simulink model "SystemModel"  (R2026a)
settings: Solver=FixedStepDiscrete  StopTime=inf  FixedStep=ts_system  EnableMultiTasking=on
StartFcn:
  | Simulink.sdi.setRecordData(false);
undefined symbols (not defined in the file): Battery, BCE12, BCE_Set_init, BMS_Controller_State, Cell10_P, Cell11_P, Cell12_P, Cell1_N, Cell1_P, Cell2_P, Cell3_P, Cell4_P, Cell5_P, Cell6_P, Cell7_P, Cell8_P, Cell9_P, Cell_Temperatures, Cell_Voltages, Charging_State, currentFactor, CV_Gain, Device_01, DiscIntNeverNeededParam, I_cc, MaxCellVoltThrsld, noCurrent, Ns_Module, NumModules, OverCellVoltageLimit, sg_bce, SOCInit, SRE, ts_controller, ts_system, UnderCellVoltageLimit, voltThreshold
libraries: slrealtimeethercatlib x99, fl_lib x65, nesl_utility x43, simulink x23, slrealtimeutilitieslib x13, sl_discontinuities x13, dspstat3 x12, canmsglib x11, speedgoatlib_IO611 x9, batt_lib x3, sharedTrackingLibrary x2, BatteryModuleLibrary_12Cells_lib x1
(part 3 of 6)

== system SystemModel/BMS/HIL ==
  note: Terminate the "Cells" Simscape Bus
  State_Request : Inport  OutDataTypeStr=Enum: SRE  PortDimensions=1
  Sensor_Values : Inport  Port=2
  Bus Creator : BusCreator  Inputs=4  OutDataTypeStr=Bus: Controller_Info  NonVirtualBus=on
      settings: InheritFromInputs=off
  Bus Creator1 : BusCreator  Inputs=4  OutDataTypeStr=Bus: Controller_Output  NonVirtualBus=on
      settings: InheritFromInputs=off
  Cell Monitoring Unit : Subsystem
  Controller : Subsystem  VariantControl=Ns_Module == 12
  Rate Transition : RateTransition  InitialCondition=struct('Cell_Voltages',3.7*ones(1,Ns_Module),'Cell_Temperatures',298.15*ones(1,Ns_Module),'Pack_Current',0,'Pack_Voltage',3.7*Ns_Module)  OutPortSampleTime=ts_controller
  Rate Transition1 : RateTransition  InitialCondition=SRE.Standby  OutPortSampleTime=ts_controller
  Simscape Bus : SimscapeBus
  Cells : PMIOPort  Side=Left
  Controller_Info : Outport
  Controller_Output : Outport  Port=2  OutDataTypeStr=Bus: Controller_Output  VectorParamsAs1DForOutWhenUnconnected=off  BusOutputAsStruct=on
  wires:
  Bus Creator/1 -> Controller_Info/1  "Controller_Info"
  Bus Creator1/1 -> Controller_Output/1  "Controller_Output"
  [Bal_Cmd_Controller] -> Cell Monitoring Unit/1(Bal_Cmd_Controller)
  Cell Monitoring Unit/1(Bal_Cmd) -> Bus Creator1/4
  Rate Transition/1 -> Cell Monitoring Unit/2(Sensor_Values)
  Cell Monitoring Unit/2(Sensor Values) -> Controller/1(Sensor_Values)
  Rate Transition1/1 -> Controller/2(State_Request)
  Controller/1(BMS_Faults) -> Bus Creator/1
  Controller/2(Charging_State) -> Bus Creator/2
  Controller/3(BMS_State) -> Bus Creator/3
  Controller/4(SOC) -> Bus Creator/4
  Controller/5(Discharge_Current_Limit) -> Bus Creator1/1
  Controller/6(Charge_Current_Limit) -> Bus Creator1/2
  Controller/7(Charge_Current_Req) -> Bus Creator1/3
  Controller/8(Bal_Cmd) -> [Bal_Cmd_Controller]
  State_Request/1 -> Rate Transition1/1
  Sensor_Values/1 -> Rate Transition/1
  connections:
  Simscape Bus/RConn1 -- Cells/RConn1

== system SystemModel/BMS/MIL ==
  State_Request : Inport  OutDataTypeStr=Enum: SRE  PortDimensions=1
  Sensor_Values : Inport  Port=2  OutDataTypeStr=Bus: Sensor_Values  BusOutputAsStruct=on
  Bus Creator : BusCreator  Inputs=4  OutDataTypeStr=Bus: Controller_Info  NonVirtualBus=on
      settings: InheritFromInputs=off
  Bus Creator1 : BusCreator  Inputs=4  OutDataTypeStr=Bus: Controller_Output  NonVirtualBus=on
      settings: InheritFromInputs=off
  Cell Monitoring Unit : Subsystem
  Controller : Subsystem
  Rate Transition : RateTransition  InitialCondition=struct('Cell_Voltages',3.7*ones(1,Ns_Module),'Cell_Temperatures',298.15*ones(1,Ns_Module),'Pack_Current',0,'Pack_Voltage',3.7*Ns_Module)  OutPortSampleTime=ts_controller
  Rate Transition1 : RateTransition  InitialCondition=SRE.Standby  OutPortSampleTime=ts_controller
  Cells : PMIOPort  Side=Left
  Controller_Info : Outport
  Controller_Output : Outport  Port=2  OutDataTypeStr=Bus: Controller_Output  VectorParamsAs1DForOutWhenUnconnected=off  BusOutputAsStruct=on
  wires:
  Bus Creator/1 -> Controller_Info/1  "Controller_Info"
  Bus Creator1/1 -> Controller_Output/1  "Controller_Output"
  State_Request/1 -> Rate Transition1/1
  Controller/1(Faults) -> Bus Creator/1
  Controller/2(Charging_State) -> Bus Creator/2  "Charging_State"
  Controller/3(BMS_Controller_State) -> Bus Creator/3  "BMS_State"
  Controller/4(SOC) -> Bus Creator/4
  Controller/5(Discharge_Current_Limit) -> Bus Creator1/1
  Controller/6(Charge_Current_Limit) -> Bus Creator1/2
  Controller/7(Charge_Current_Req) -> Bus Creator1/3
  Controller/8(Bal_Cmd) -> [Bal_Cmd_Controller]
  [Bal_Cmd_Controller] -> Cell Monitoring Unit/1(Bal_Cmd_Controller)
  Sensor_Values/1 -> Rate Transition/1
  Cell Monitoring Unit/1(Bal_Cmd) -> Bus Creator1/4
  Cell Monitoring Unit/2(Sensor Values) -> Controller/1(Sensor_Values)
  Rate Transition1/1 -> Controller/2(State_Request)
  Rate Transition/1 -> Cell Monitoring Unit/2(Sensor_Values)
  connections:
  Cells/RConn1 -- Cell Monitoring Unit/LConn1

== system SystemModel/Battery/Battery Pack ==
  Ambient_Temperature : Inport
  Short_Circuits : Inport  Port=2
  12-Cell : Subsystem  VariantControl=Ns_Module == 12
  Batt+ : PMIOPort  Side=Right
  Batt- : PMIOPort  Port=2  Side=Right
  Cells : PMIOPort  Port=3  Side=Right
  Cell_Voltages : Outport
  Cell_Temperatures : Outport  Port=2
  Cell_SOCs : Outport  Port=3
  wires:
  Ambient_Temperature/1 -> 12-Cell/1(Ambient_Temperature)
  Short_Circuits/1 -> 12-Cell/2(Short_Circuits)
  12-Cell/1(Cell_Voltages) -> Cell_Voltages/1
  12-Cell/2(Cell_Temperatures) -> Cell_Temperatures/1
  12-Cell/3(Cell_SOCs) -> Cell_SOCs/1
  connections:
  12-Cell/RConn1 -- Batt+/RConn1
  12-Cell/RConn2 -- Batt-/RConn1
  12-Cell/RConn3 -- Cells/RConn1

== system SystemModel/Battery/Bypass ==
  IN : Inport
  Bus Assignment : BusAssignment  AssignedSignals=Cell_Voltages,Cell_Temperatures
  Bus Selector : BusSelector  OutputSignals=Cell_Voltages,Cell_Temperatures
  Bypass Values : Subsystem
  Data Type Conversion{,1..3} (4 alike) : DataTypeConversion  OutDataTypeStr=single  SaturateOnIntegerOverflow=off  RndMeth=Floor
  OUT : Outport
  wires:
  IN/1 -> Bus Assignment/1, Bus Selector/1
  Bus Assignment/1 -> OUT/1
  [Cell_Voltages_OUT] -> Data Type Conversion/1
  [Cell_Temperatures_OUT] -> Data Type Conversion1/1
  Bus Selector/1 -> [Cell_Voltages_IN]  "<Cell_Voltages>"
  Bus Selector/2 -> [Cell_Temperatures_IN]  "<Cell_Temperatures>"
  Data Type Conversion/1 -> Bus Assignment/2
  Data Type Conversion1/1 -> Bus Assignment/3
  Data Type Conversion2/1 -> [Cell_Voltages_OUT]
  Data Type Conversion3/1 -> [Cell_Temperatures_OUT]
  [Cell_Voltages_IN] -> Bypass Values/1(Input_Voltages)
  [Cell_Temperatures_IN] -> Bypass Values/2(Input_Temperatures)
  Bypass Values/1(Output_Voltages) -> Data Type Conversion2/1
  Bypass Values/2(Output_Temperatures) -> Data Type Conversion3/1
  [Broken_Wires_User] -> Bypass Values/3(Broken_Wire)

== system SystemModel/Battery/Electrical Interface ==
  Current_Request : Inport
  Controlled Current Source : fl_lib/Electrical/Electrical Sources/Controlled Current Source
  Current Sensor : fl_lib/Electrical/Electrical Sensors/Current Sensor
  Data Type Conversion : DataTypeConversion  OutDataTypeStr=double  SaturateOnIntegerOverflow=off  RndMeth=Floor
  Electrical Reference : fl_lib/Electrical/Electrical Elements/Electrical Reference
  PS-Simulink Converter : nesl_utility/PS-Simulink Converter  PhysicalDomain=network_engine_domain  SubClassName=ps_output  LeftPortType=input  RightPortType=output  PseudoPeriodic=off  Frequencies=[]  VectorFormat=inherit  Unit=inherit  AffineConversion=off
  PS-Simulink Converter1 : nesl_utility/PS-Simulink Converter  PhysicalDomain=network_engine_domain  SubClassName=ps_output  LeftPortType=input  RightPortType=output  PseudoPeriodic=off  Frequencies=[]  VectorFormat=inherit  Unit=inherit  AffineConversion=off
  Simulink-PS Converter3 : nesl_utility/Simulink-PS Converter  PhysicalDomain=network_engine_domain  SubClassName=ps_input  LeftPortType=input  RightPortType=output  PseudoPeriodic=off  Frequencies=[]  NoiseDistribution=none  NoiseParameters=[]  Unit=1  AffineConversion=off  FilteringAndDerivatives=zero  SimscapeFilterOrder=1  InputFilterTimeConstant=0.001  UdotUserProvided=1
  Solver Configuration : nesl_utility/Solver Configuration  PhysicalDomain=network_engine_domain  SubClassName=solver  LeftPortType=input  RightPortType=generic  Tones=[]  Harmonics=[]  SimulateNoise=off  Profile=off  UseLocalSampling=off  EnableSwitchedLinearOptims=on  FrequencyDomain=off  UseCCode=off  RelTol=0.001  AbsTol=0.001  MinStep=1e-09  ToWorkspace=off  RevertToSquareIcSolve=off  NumHomotopyIterations=100  PhasorMode=off  PhasorModeNumHarmonics=1  ConsistencySolver=NEWTON_XTOL_AFTER_FTOL  CanonicalOrdering=UNORDERED  OptimizeIntermediates=UNOPTIMIZED  IndexReductionMethod=DerivativeReplacement  DoDC=off  ResidualTolerance=1e-09  ConsistencyTolSource=GLOBAL  ConsistencyAbsTol=0.001  ConsistencyRelTol=0.001  ConsistencyTolFactor=1e-09  UseLocalSolver=on  LocalSolverChoice=NE_BACKWARD_EULER_ADVANCER  ResolveIndetEquations=on  FunctionEvalNumThread=1  LocalSolverSampleTime=ts_system  DoFixedCost=on  MaxNonlinIter=3  MaxModeIter=2  ComputeImpulses=off  ImpulseIterations=2  LinearAlgebra=auto  LinearAlgebraNumThread=0  EquationFormulation=NE_TIME_EF  DelaysMemoryBudget=1024  AutomaticFiltering=on  FilteringTimeConstant=0.001  PartitionStorageMethod=AS_NEEDED  PartitionMemoryBudget=1024  PartitionMethod=ROBUST  MultibodyUseLocalSolver=off  MultibodyLocalSolverChoice=ODE1  MultibodyLocalSolverSampleTime=0.001
  Voltage Sensor7 : fl_lib/Electrical/Electrical Sensors/Voltage Sensor
      settings: LibrarySourceBlock=BatteryPack_lib/CellMonitoringUnit/Voltage Sensor1
  Batt+ : PMIOPort  Side=Left
  Batt- : PMIOPort  Port=2  Side=Left
  Pack_Current : Outport
  Pack_Voltage : Outport  Port=2
  wires:
  Current_Request/1 -> Data Type Conversion/1
  PS-Simulink Converter1/1 -> Pack_Current/1
  PS-Simulink Converter/1 -> Pack_Voltage/1
  Data Type Conversion/1 -> Simulink-PS Converter3/1
  connections:
  Controlled Current Source/LConn1 -- Voltage Sensor7/LConn1 -- Batt+/RConn1
  Current Sensor/RConn2 -- Solver Configuration/RConn1 -- Electrical Reference/LConn1 -- Controlled Current Source/RConn2
  PS-Simulink Converter1/LConn1 -- Current Sensor/RConn1
  Simulink-PS Converter3/RConn1 -- Controlled Current Source/RConn1
  Batt-/RConn1 -- Voltage Sensor7/RConn2 -- Current Sensor/LConn1
  Voltage Sensor7/RConn1 -- PS-Simulink Converter/LConn1

== system SystemModel/Battery/HW Interface ==
  Sensor_Values_Sim : Inport
  BCE - HIL : Subsystem  VariantControl=strcmp(get_param([bdroot '/Instrumentation/Simulation_Profile_Value'], 'Value'),'1') && Ns_Module == 12
  MIL : Subsystem  VariantControl=strcmp(get_param([bdroot '/Instrumentation/Simulation_Profile_Value'], 'Value'),'0')
  Cells_IN : PMIOPort  Side=Left
  Cells_OUT : PMIOPort  Port=2  Side=Right
  Sensor_Values_Real : Outport

== system SystemModel/Instrumentation/Celsius_to_Kelvin ==
  C : Inport
  Add : Sum
  Constant4 : Constant  Value=273.15
  K : Outport
  wires:
  Constant4/1 -> Add/2
  C/1 -> Add/1
  Add/1 -> K/1

== system SystemModel/Instrumentation/Current Control ==
  Current_Request_User : Inport
  Current_Request_User_Bypass : Inport  Port=2
  Controller_Info : Inport  Port=3
  Controller_Output : Inport  Port=4
  Bus Selector : BusSelector  OutputSignals=Charge_Current_Limit,Discharge_Current_Limit
  Bus Selector1 : BusSelector  OutputSignals=BMS_State
  Compare To Constant : simulink/Logic and Bit Operations/Compare To Constant  relop===  const=BMS_Controller_State.BMS_Fault  OutDataTypeStr=uint8
  Current_Req : Constant  Value=0  SampleTime=ts_controller
  Saturation Dynamic : sl_discontinuities/Saturation Dynamic  OutMin=[]  OutMax=[]  OutDataTypeStr=Inherit: Same as second input  OutDataType=fixdt(1, 16)  OutScaling=2^-10  DoSatur=off
  Switch : Switch  Criteria=u2 > Threshold  SaturateOnIntegerOverflow=off  InputSameDT=off
  Switch1 : Switch  Criteria=u2 > Threshold  SaturateOnIntegerOverflow=off  InputSameDT=off
  Current_Request : Outport
  wires:
  Current_Request_User/1 -> Saturation Dynamic/2, Switch1/1
  Controller_Output/1 -> Bus Selector/1
  Bus Selector/1 -> Saturation Dynamic/1  "<Charge_Current_Limit>"
  Bus Selector/2 -> Saturation Dynamic/3  "<Discharge_Current_Limit>"
  Current_Req/1 -> Switch/1
  Saturation Dynamic/1 -> Switch/3
  Controller_Info/1 -> Bus Selector1/1
  Bus Selector1/1 -> Compare To Constant/1  "<BMS_State>"
  Switch1/1 -> Current_Request/1
  Switch/1 -> Switch1/3
  Current_Request_User_Bypass/1 -> Switch1/2
  Compare To Constant/1 -> Switch/2

== system SystemModel/Instrumentation/Instrumented Signals ==
  Controller_Output : Inport
  Controller_Info : Inport  Port=2
  Sensor_Values : Inport  Port=3
  Balancing_Currents : Inport  Port=4
  Cells_SOCs : Inport  Port=5
  12-Cell : Subsystem  VariantControl=Ns_Module == 12
  Short-Circuits : Outport
  Broken_Wires : Outport  Port=2
  wires:
  Controller_Output/1 -> 12-Cell/1(Controller_Output)
  Controller_Info/1 -> 12-Cell/2(Controller_Info)
  Sensor_Values/1 -> 12-Cell/3(Sensor_Values)
  Balancing_Currents/1 -> 12-Cell/4(Balancing_Currents)
  Cells_SOCs/1 -> 12-Cell/5(Cells_SOCs)
  12-Cell/1(Short-Circuits) -> Short-Circuits/1
  12-Cell/2(Broken_Wires) -> Broken_Wires/1

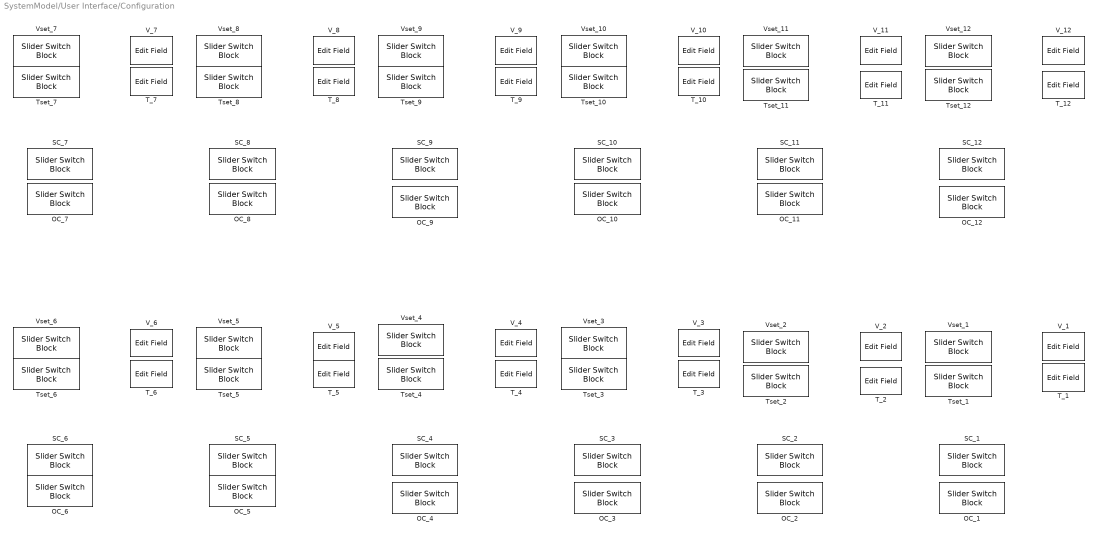
== system SystemModel/User Interface/Configuration ==
  OC_{1..12} (12 alike) : SliderSwitchBlock  LabelPosition=Hide
  SC_{1..12} (12 alike) : SliderSwitchBlock  LabelPosition=Hide
  T_{1..12} (12 alike) : EditField  LabelPosition=Hide  ShowInitialText=on  Alignment=Center
  Tset_{1..12} (12 alike) : SliderSwitchBlock  LabelPosition=Hide
  V_{1..12} (12 alike) : EditField  LabelPosition=Hide  ShowInitialText=on  Alignment=Center
  Vset_{1..12} (12 alike) : SliderSwitchBlock  LabelPosition=Hide

== system SystemModel/BMS/HIL/Cell Monitoring Unit ==
  Bal_Cmd_Controller : Inport
  Sensor_Values : Inport  Port=2
  Bal_Cmd : Outport
  Sensor Values : Outport  Port=2
  wires:
  Sensor_Values/1 -> Sensor Values/1
  Bal_Cmd_Controller/1 -> Bal_Cmd/1  "Bal_Cmd"

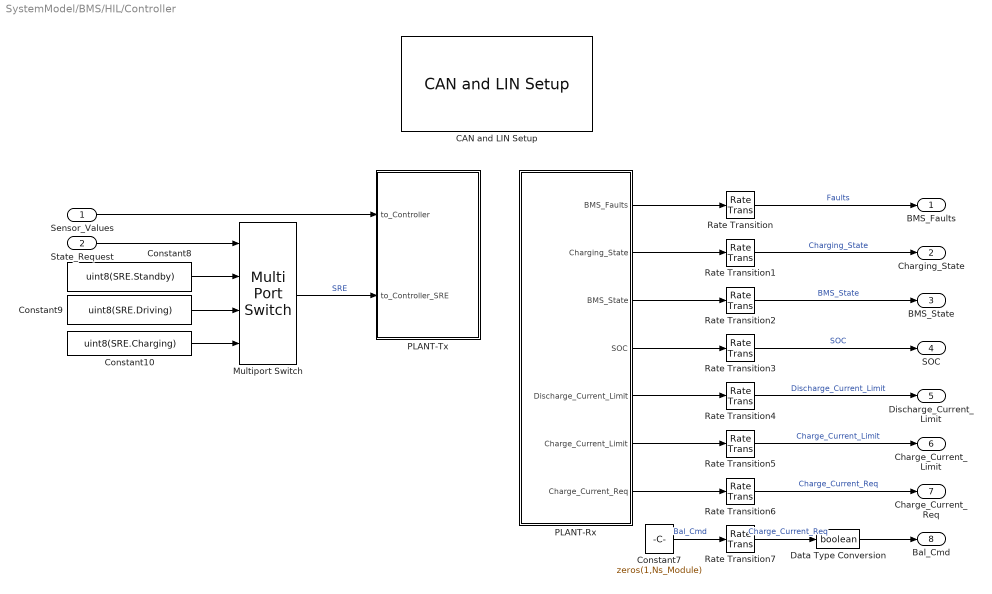
== system SystemModel/BMS/HIL/Controller ==
  Sensor_Values : Inport  OutDataTypeStr=Bus: Sensor_Values  BusOutputAsStruct=on
  State_Request : Inport  Port=2  OutDataTypeStr=Enum: SRE  PortDimensions=1
  "CAN and LIN Setup " : speedgoatlib_IO611/CAN and LIN Setup   moduleInitValues="[611    1    1   -1   -1]"  id=1  moduleType=IO611  pciSlot=-1  canChn1=CAN (HS)  canChn2=CAN (HS)  canChn3=Disabled  canChn4=Disabled  linChn1=Disabled  linChn2=Disabled  canInitStructArray=[]  canTermStructArray=[]  canChn1InitValues="[2   2   1  31   8   2   1   5   2]"  arbBdrChn1=1.0 MBaud  arbManBdrChn1=[2,1,31,8]  fdBdrChn1=5.0 MBaud  fdManBdrChn1=[2,1,5,2]  canChn2InitValues="[2   2   1  31   8   2   1   5   2]"  arbBdrChn2=1.0 MBaud  arbManBdrChn2=[2,1,31,8]  fdBdrChn2=5.0 MBaud  fdManBdrChn2=[2,1,5,2]  canChn3InitValues="[1   2   1  31   8   2   1   5   2]"  arbBdrChn3=1.0 MBaud  arbManBdrChn3=[2,1,31,8]  fdBdrChn3=5.0 MBaud  fdManBdrChn3=[2,1,5,2]  canChn4InitValues="[1   2   1  31   8   2   1   5   2]"  arbBdrChn4=1.0 MBaud  arbManBdrChn4=[2,1,31,8]  fdBdrChn4=5.0 MBaud  fdManBdrChn4=[2,1,5,2]  bdrLIN1=19200  linChn1InitValues="[1  19200]"  bdrLIN2=19200  linChn2InitValues="[1  19200]"
      settings: LibrarySourceBlock=speedgoatlib_CANLIN_OfA2/CAN and LIN Setup
  Constant10 : Constant  Value=uint8(SRE.Charging)
  Constant7 : Constant  Value=zeros(1,Ns_Module)
  Constant8 : Constant  Value=uint8(SRE.Standby)
  Constant9 : Constant  Value=uint8(SRE.Driving)
  Data Type Conversion : DataTypeConversion  OutDataTypeStr=boolean  SaturateOnIntegerOverflow=off  RndMeth=Floor
  Multiport Switch : MultiPortSwitch  DataPortOrder=Specify indices  DataPortIndices={SRE.Standby, SRE.Driving, SRE.Charging}  SaturateOnIntegerOverflow=off  InputSameDT=off
  PLANT-Rx : Subsystem  TreatAsAtomicUnit=on
  PLANT-Tx : Subsystem
  Rate Transition : RateTransition  InitialCondition=struct('OverCurrent',0,'HighTemp',0,'LowTemp',0,'OverVolt',0,'UnderVolt',0)  OutPortSampleTime=ts_controller
  Rate Transition1 : RateTransition  InitialCondition=Charging_State.Init  OutPortSampleTime=ts_controller
  Rate Transition2 : RateTransition  InitialCondition=BMS_Controller_State.BMS_Idle  OutPortSampleTime=ts_controller
  Rate Transition3 : RateTransition  InitialCondition=[0, 0, 0]  OutPortSampleTime=ts_controller
  Rate Transition4 : RateTransition  InitialCondition=-100  OutPortSampleTime=ts_controller
  Rate Transition5 : RateTransition  InitialCondition=40  OutPortSampleTime=ts_controller
  Rate Transition6 : RateTransition  OutPortSampleTime=ts_controller
  Rate Transition7 : RateTransition  OutPortSampleTime=ts_controller
  BMS_Faults : Outport
  Charging_State : Outport  Port=2
  BMS_State : Outport  Port=3
  SOC : Outport  Port=4
  Discharge_Current_Limit : Outport  Port=5
  Charge_Current_Limit : Outport  Port=6
  Charge_Current_Req : Outport  Port=7
  Bal_Cmd : Outport  Port=8
  wires:
  Constant7/1 -> Rate Transition7/1  "Bal_Cmd"
  Constant9/1 -> Multiport Switch/3
  Constant10/1 -> Multiport Switch/4
  Constant8/1 -> Multiport Switch/2
  State_Request/1 -> Multiport Switch/1
  PLANT-Rx/1(BMS_Faults) -> Rate Transition/1
  PLANT-Rx/7(Charge_Current_Req) -> Rate Transition6/1
  PLANT-Rx/6(Charge_Current_Limit) -> Rate Transition5/1
  PLANT-Rx/5(Discharge_Current_Limit) -> Rate Transition4/1
  PLANT-Rx/4(SOC) -> Rate Transition3/1
  PLANT-Rx/3(BMS_State) -> Rate Transition2/1
  PLANT-Rx/2(Charging_State) -> Rate Transition1/1
  Rate Transition/1 -> BMS_Faults/1  "Faults"
  Rate Transition1/1 -> Charging_State/1  "Charging_State"
  Rate Transition2/1 -> BMS_State/1  "BMS_State"
  Rate Transition3/1 -> SOC/1  "SOC"
  Rate Transition4/1 -> Discharge_Current_Limit/1  "Discharge_Current_Limit"
  Rate Transition5/1 -> Charge_Current_Limit/1  "Charge_Current_Limit"
  Rate Transition6/1 -> Charge_Current_Req/1  "Charge_Current_Req"
  Data Type Conversion/1 -> Bal_Cmd/1
  Rate Transition7/1 -> Data Type Conversion/1  "Charge_Current_Req"
  Sensor_Values/1 -> PLANT-Tx/1(to_Controller)
  Multiport Switch/1 -> PLANT-Tx/2(to_Controller_SRE)  "SRE"

== system SystemModel/BMS/MIL/Cell Monitoring Unit ==
  Bal_Cmd_Controller : Inport
  Sensor_Values : Inport  Port=2
  Balancing_Circuit : Subsystem
  Feedback Unit : UnitDelay  InitialCondition=struct('Cell_Voltages',3.6*ones(1, Ns_Module*NumModules),'Cell_Temperatures',293.15*ones(1,Ns_Module*NumModules),'Pack_Current',0,'Pack_Voltage',3.6*Ns_Module*NumModules)  SampleTime=-1
  Rate Transition1 : RateTransition  InitialCondition=zeros(1,Ns_Module)  OutPortSampleTime=ts_system
  Cells : PMIOPort  Side=Left
  Bal_Cmd : Outport
  Sensor Values : Outport  Port=2
  tag scope: Balancing_Currents=global
  wires:
  Feedback Unit/1 -> Sensor Values/1
  Sensor_Values/1 -> Feedback Unit/1
  Bal_Cmd_Controller/1 -> Bal_Cmd/1, Rate Transition1/1
  Rate Transition1/1 -> Balancing_Circuit/1(Bal_Cmd_Controller)
  Balancing_Circuit/1(Balancing_Currents) -> [Balancing_Currents]
  connections:
  Balancing_Circuit/LConn1 -- Cells/RConn1

== system SystemModel/BMS/MIL/Controller ==
  Sensor_Values : Inport  OutDataTypeStr=Bus: Sensor_Values  BusOutputAsStruct=on
  State_Request : Inport  Port=2  OutDataTypeStr=Enum: SRE  PortDimensions=1
  BMS State Machine : Subsystem
  Balancing Logic : Subsystem
  Constant : Constant
  Current Calculations : Subsystem
  SOC Calculation : Subsystem
  Faults : Outport
  Charging_State : Outport  Port=2
  BMS_Controller_State : Outport  Port=3
  SOC : Outport  Port=4
  Discharge_Current_Limit : Outport  Port=5
  Charge_Current_Limit : Outport  Port=6
  Charge_Current_Req : Outport  Port=7
  Bal_Cmd : Outport  Port=8
  wires:
  SOC Calculation/1(SOC) -> SOC/1
  Current Calculations/1(Discharge_Current_Limit) -> Discharge_Current_Limit/1, BMS State Machine/1(Discharge_Current_Limit)
  BMS State Machine/2(Faults) -> Faults/1
  BMS State Machine/1(Charge_Current_Req) -> Charge_Current_Req/1
  Sensor_Values/1 -> Balancing Logic/2(Sensor_Values), SOC Calculation/2(Sensor_Values), BMS State Machine/4(Sensor_Values), Current Calculations/1(BMS_Input)
  BMS State Machine/4(BMS_State) -> BMS_Controller_State/1, Balancing Logic/1(BMS_State), SOC Calculation/1(BMS_State)
  Current Calculations/2(Charge_Current_Limit) -> Charge_Current_Limit/1, BMS State Machine/2(Charge_Current_Limit)
  Balancing Logic/1(Bal_Cmd) -> Bal_Cmd/1  "Bal_Cmd"
  State_Request/1 -> BMS State Machine/3(State_Request)
  Constant/1 -> BMS State Machine/5(Fault_Reset_Enable)
  BMS State Machine/3(Charging_State) -> Charging_State/1

== system SystemModel/Battery/Battery Pack/12-Cell ==
  Ambient_Temperature : Inport
  Short_Circuits : Inport  Port=2
  Controlled Temperature Source : fl_lib/Thermal/Thermal Sources/Controlled Temperature Source
      settings: LibrarySourceBlock=|
      | BatteryPack_lib/CellModule1TC/Controlled
      | Temperature Source
  Delay : Delay
  Faults : Subsystem
  Module1 : BatteryModuleLibrary_12Cells_lib/Module1  BatteryCapacityCell=27 A*hr  ExtrapolationMethodCell=simscape.enum.extrapolation.nearest  SOCBreakpointsCell=[0, .1, .25, .5, .75, .9, 1]  TemperatureBreakpointsCell=[278, 293, 313] K  OpenCircuitVoltageThermalCell=[3.49, 3.5, 3.51; 3.55, 3.57, 3.56; 3.62, 3.63, 3.64; 3.71, 3.71, 3.72; 3.91, 3.93, 3.94; 4.07, 4.08, 4.08; 4.19, 4.19, 4.19] V  VoltageRangeCell=[0, inf] V  ResistanceSOCBreakpointsCell=[0, .1, .25, .5, .75, .9, 1]  ResistanceTemperatureBreakpointsCell=[278, 293, 313] K  R0ThermalCell=[.0117, .0085, .009; .011, .0085, .009; .0114, .0087, .0092; .0107, .0082, .0088; .0107, .0083, .0091; .0113, .0085, .0089; .0116, .0085, .0089] Ohm  BatteryThermalMassCell=100 J/K  AmbientResistance=25 K/W  P=1  S=12  socCell_specify=off  socCell_priority=High  socCell=repmat(1, 12, 1)  socCell_nominal_specify=off  socCell_nominal_value=1  socCell_nominal_unit=1  numCycles_specify=off  numCycles_priority=High  numCycles=repmat(0, 12, 1)  numCycles_nominal_specify=off  numCycles_nominal_value=1  numCycles_nominal_unit=1  batteryVoltage_specify=off  batteryVoltage_priority=None  batteryVoltage=repmat(0, 12, 1) V  batteryVoltage_nominal_specify=off  batteryVoltage_nominal_value=1  batteryVoltage_nominal_unit=V  batteryCurrent_specify=off  batteryCurrent_priority=None  batteryCurrent=repmat(0, 12, 1) A  batteryCurrent_nominal_specify=off  batteryCurrent_nominal_value=1  batteryCurrent_nominal_unit=A  batteryTemperature_specify=off  batteryTemperature_priority=High  batteryTemperature=repmat(298.15, 12, 1) K  batteryTemperature_nominal_specify=off  batteryTemperature_nominal_value=1  batteryTemperature_nominal_unit=K  vParallelAssembly_specify=off  vParallelAssembly_priority=None  vParallelAssembly=repmat(0, 12, 1) V  vParallelAssembly_nominal_specify=off  vParallelAssembly_nominal_value=1  vParallelAssembly_nominal_unit=V  socParallelAssembly_specify=off  socParallelAssembly_priority=None  socParallelAssembly=repmat(1, 12, 1)  socParallelAssembly_nominal_specify=off  socParallelAssembly_nominal_value=1  socParallelAssembly_nominal_unit=1
  PS-Simulink Converter : nesl_utility/PS-Simulink Converter  PhysicalDomain=network_engine_domain  SubClassName=ps_output  LeftPortType=input  RightPortType=output  PseudoPeriodic=off  Frequencies=[]  VectorFormat=inherit  Unit=inherit  AffineConversion=off
  Passive Balancing Interface : batt_lib/HIL/Passive Balancing Interface  balancingCircuitCount=12
  Probe : SimscapeProbe  BoundBlock=23330  Variables={batteryTemperature, socParallelAssembly}
  Simulink-PS Converter : nesl_utility/Simulink-PS Converter  PhysicalDomain=network_engine_domain  SubClassName=ps_input  LeftPortType=input  RightPortType=output  PseudoPeriodic=off  Frequencies=[]  NoiseDistribution=none  NoiseParameters=[]  Unit=1  AffineConversion=off  FilteringAndDerivatives=provide  SimscapeFilterOrder=1  InputFilterTimeConstant=0.001  UdotUserProvided=0
  Simulink-PS Converter1 : nesl_utility/Simulink-PS Converter  PhysicalDomain=network_engine_domain  SubClassName=ps_input  LeftPortType=input  RightPortType=output  PseudoPeriodic=off  Frequencies=[]  NoiseDistribution=none  NoiseParameters=[]  Unit=1  AffineConversion=off  FilteringAndDerivatives=provide  SimscapeFilterOrder=1  InputFilterTimeConstant=0.001  UdotUserProvided=0
      settings: LibrarySourceBlock=|
      | BatteryPack_lib/CellModule1TC/Simulink-PS
      | Converter1
  Batt+ : PMIOPort  Side=Right
  Batt- : PMIOPort  Port=2  Side=Right
  Cells : PMIOPort  Port=3  Side=Right
  Cell_Voltages : Outport
  Cell_Temperatures : Outport  Port=2
  Cell_SOCs : Outport  Port=3
  wires:
  [Balancing_Currents] -> Delay/1
  Probe/1 -> Cell_Temperatures/1
  Probe/2 -> Cell_SOCs/1
  Delay/1 -> Simulink-PS Converter/1
  Short_Circuits/1 -> Faults/1(Short_Circuits)
  Ambient_Temperature/1 -> Simulink-PS Converter1/1
  PS-Simulink Converter/1 -> Cell_Voltages/1
  connections:
  Controlled Temperature Source/LConn1 -- Module1/LConn1
  Batt+/RConn1 -- Module1/LConn2
  Batt-/RConn1 -- Module1/RConn3
  Passive Balancing Interface/LConn1 -- Module1/RConn1 -- Faults/RConn1
  Passive Balancing Interface/RConn1 -- Simulink-PS Converter/RConn1
  PS-Simulink Converter/LConn1 -- Passive Balancing Interface/RConn2
  Module1/RConn2 -- Passive Balancing Interface/LConn2 -- Faults/RConn3
  Cells/RConn1 -- Faults/RConn2
  Simulink-PS Converter1/RConn1 -- Controlled Temperature Source/RConn1

== system SystemModel/Battery/Bypass/Bypass Values ==
  Input_Voltages : Inport
  Input_Temperatures : Inport  Port=2
  Broken_Wire : Inport  Port=3
  12-Cell : Subsystem  VariantControl=Ns_Module == 12
  Output_Voltages : Outport
  Output_Temperatures : Outport  Port=2
  wires:
  Input_Voltages/1 -> 12-Cell/1(Input_Voltages)
  Input_Temperatures/1 -> 12-Cell/2(Input_Temperatures)
  12-Cell/1(Output_Voltages) -> Output_Voltages/1
  12-Cell/2(Output_Temperatures) -> Output_Temperatures/1
  Broken_Wire/1 -> 12-Cell/3(Broken_Wire)

== system SystemModel/Battery/HW Interface/BCE - HIL ==
  Sensor_Values_Sim : Inport
  Add : Sum  Inputs=+
  Battery Cell Emulator : Subsystem
  Bus Creator : BusCreator  Inputs=4  OutDataTypeStr=Bus: Sensor_Values  NonVirtualBus=on
      settings: InheritFromInputs=off
  Data Type Conversion : DataTypeConversion  SaturateOnIntegerOverflow=off  RndMeth=Floor
  Shunt Emulator : Subsystem
  Temperature Emulator : Subsystem
  Cells_IN : PMIOPort  Side=Left
  Cells_OUT : PMIOPort  Port=2  Side=Right
  Sensor_Values_Real : Outport
  tag scope: Balancing_Currents=global
  wires:
  Sensor_Values_Sim/1 -> Battery Cell Emulator/1(Sensor_Values_Sim), Shunt Emulator/1(Sensor_Values_Sim), Temperature Emulator/1(Sensor_Values_Sim)
  Battery Cell Emulator/2(Cell_Voltages) -> Bus Creator/1, Add/1  "Cell_Voltages"
  Temperature Emulator/1(Cell_Temperatures) -> Bus Creator/2  "Cell_Temperatures"
  Add/1 -> Bus Creator/4  "Pack_Voltage"
  Bus Creator/1 -> Sensor_Values_Real/1
  Shunt Emulator/1(Pack_Current) -> Bus Creator/3  "Pack_Current"
  Battery Cell Emulator/1(Current_Values) -> Data Type Conversion/1
  Data Type Conversion/1 -> [Balancing_Currents]
  connections:
  Cells_OUT/RConn1 -- Cells_IN/RConn1

== system SystemModel/Battery/HW Interface/MIL ==
  Sensor_Values_Sim : Inport
  Cells_IN : PMIOPort  Side=Left
  Cells_OUT : PMIOPort  Port=2  Side=Right
  Sensor_Values_Real : Outport
  wires:
  Sensor_Values_Sim/1 -> Sensor_Values_Real/1
  connections:
  Cells_IN/RConn1 -- Cells_OUT/RConn1

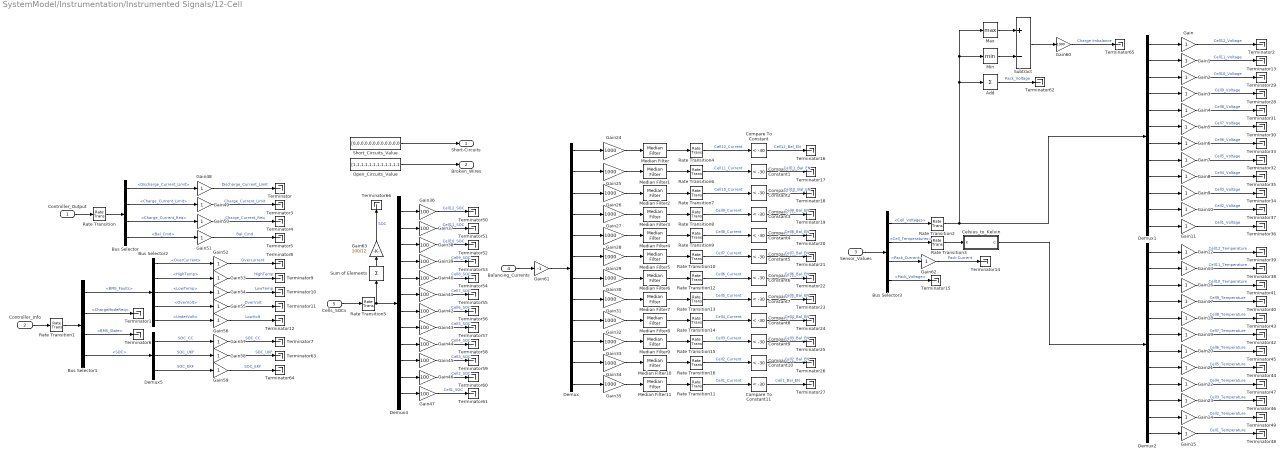
== system SystemModel/Instrumentation/Instrumented Signals/12-Cell ==
  Controller_Output : Inport
  Controller_Info : Inport  Port=2
  Sensor_Values : Inport  Port=3
  Balancing_Currents : Inport  Port=4
  Cells_SOCs : Inport  Port=5
  Add : Sum  Inputs=+
  Bus Selector : BusSelector  OutputSignals=Discharge_Current_Limit,Charge_Current_Limit,Charge_Current_Req,Bal_Cmd
  Bus Selector1 : BusSelector  OutputSignals=BMS_Faults,ChargeModeReq,BMS_State,SOC
  Bus Selector2 : BusSelector  OutputSignals=OverCurrent,HighTemp,LowTemp,OverVolt,UnderVolt
  Bus Selector3 : BusSelector  OutputSignals=Cell_Voltages,Cell_Temperatures,Pack_Current,Pack_Voltage
  Celsius_to_Kelvin : Subsystem
  Compare To Constant{,1..11} (12 alike) : simulink/Logic and Bit Operations/Compare To Constant  relop=<  const=-30  OutDataTypeStr=boolean
  Demux{,1..2,4} (4 alike) : Demux  Outputs=12
  Demux5 : Demux  Outputs=3
  Gain{,1..23,48..51,57..59} (31 alike) : Gain
  Gain{24..35,60} (13 alike) : Gain  Gain=1000
  Gain{36..47} (12 alike) : Gain  Gain=100
  Gain{52..56,62} (6 alike) : Gain  OutDataTypeStr=single
  Gain61 : Gain  Gain=-1
  Gain63 : Gain  Gain=100/12
  Max : MinMax  Function=max
  Median Filter{,1..11} (12 alike) : dspstat3/Median Filter  WindowLength=7  SimulateUsing=Code generation
  Min : MinMax
  Open_Circuits_Value : Constant  Value=[1,1,1,1,1,1,1,1,1,1,1,1]
  Rate Transition{,1..16} (17 alike) : RateTransition  OutPortSampleTime=0.1
  Short_Circuits_Value : Constant  Value=[0,0,0,0,0,0,0,0,0,0,0,0]
  Subtract : Sum  Inputs=+-
  Sum of Elements : Sum  Inputs=+
  Terminator{,1..66} (67 alike) : Terminator
  Short-Circuits : Outport
  Broken_Wires : Outport  Port=2
  wires:
  Controller_Output/1 -> Rate Transition/1
  Controller_Info/1 -> Rate Transition1/1
  Sensor_Values/1 -> Bus Selector3/1
  Bus Selector/1 -> Gain48/1  "<Discharge_Current_Limit>"
  Bus Selector/2 -> Gain49/1  "<Charge_Current_Limit>"
  Bus Selector/3 -> Gain50/1  "<Charge_Current_Req>"
  Bus Selector/4 -> Gain51/1  "<Bal_Cmd>"
  Rate Transition/1 -> Bus Selector/1
  Bus Selector1/2 -> Terminator1/1  "<ChargeModeReq>"
  Bus Selector1/3 -> Terminator6/1  "<BMS_State>"
  Bus Selector1/4 -> Demux5/1  "<SOC>"
  Bus Selector2/1 -> Gain52/1  "<OverCurrent>"
  Bus Selector2/2 -> Gain53/1  "<HighTemp>"
  Bus Selector2/3 -> Gain54/1  "<LowTemp>"
  Bus Selector2/4 -> Gain55/1  "<OverVolt>"
  Bus Selector2/5 -> Gain56/1  "<UnderVolt>"
  Rate Transition1/1 -> Bus Selector1/1
  Bus Selector3/1 -> Rate Transition2/1  "<Cell_Voltages>"
  Bus Selector3/2 -> Rate Transition3/1  "<Cell_Temperatures>"
  Bus Selector3/3 -> Gain62/1  "<Pack_Current>"
  Bus Selector3/4 -> Terminator15/1  "<Pack_Voltage>"
  Demux/1 -> Gain24/1
  Demux/2 -> Gain25/1
  Demux/3 -> Gain26/1
  Demux/6 -> Gain29/1
  Demux/5 -> Gain28/1
  Demux/4 -> Gain27/1
  Demux/9 -> Gain32/1
  Demux/11 -> Gain34/1
  Demux/7 -> Gain30/1
  Demux/8 -> Gain31/1
  Demux/10 -> Gain33/1
  Demux/12 -> Gain35/1
  Rate Transition2/1 -> Add/1, Min/1, Max/1, Demux1/1
  Balancing_Currents/1 -> Gain61/1
  Demux1/1 -> Gain/1
  Demux1/2 -> Gain1/1
  Demux1/4 -> Gain3/1
  Demux1/3 -> Gain2/1
  Demux1/6 -> Gain5/1
  Demux1/7 -> Gain6/1
  Demux1/8 -> Gain7/1
  Demux1/5 -> Gain4/1
  Demux1/10 -> Gain9/1
  Demux1/11 -> Gain10/1
  Demux1/12 -> Gain11/1
  Demux1/9 -> Gain8/1
  Gain/1 -> Terminator2/1  "Cell12_Voltage"
  Gain1/1 -> Terminator13/1  "Cell11_Voltage"
  Gain2/1 -> Terminator29/1  "Cell10_Voltage"
  Gain3/1 -> Terminator28/1  "Cell9_Voltage"
  Gain4/1 -> Terminator31/1  "Cell8_Voltage"
  Gain5/1 -> Terminator30/1  "Cell7_Voltage"
  Gain6/1 -> Terminator33/1  "Cell6_Voltage"
  Gain7/1 -> Terminator32/1  "Cell5_Voltage"
  Gain8/1 -> Terminator35/1  "Cell4_Voltage"
  Gain9/1 -> Terminator34/1  "Cell3_Voltage"
  Gain10/1 -> Terminator37/1  "Cell2_Voltage"
  Gain11/1 -> Terminator36/1  "Cell1_Voltage"
  Gain22/1 -> Terminator47/1  "Cell4_Temperature"
  Gain19/1 -> Terminator42/1  "Cell7_Temperature"
  Gain17/1 -> Terminator40/1  "Cell9_Temperature"
  Gain13/1 -> Terminator38/1  "Cell11_Temperature"
  Demux2/10 -> Gain23/1
  Demux2/12 -> Gain15/1
  Demux2/11 -> Gain14/1
  Demux2/9 -> Gain22/1
  Demux2/2 -> Gain13/1
  Gain14/1 -> Terminator49/1  "Cell2_Temperature"
  Demux2/3 -> Gain16/1
  Demux2/4 -> Gain17/1
  Demux2/1 -> Gain12/1
  Gain20/1 -> Terminator45/1  "Cell6_Temperature"
  Gain12/1 -> Terminator39/1  "Cell12_Temperature"
  Gain16/1 -> Terminator41/1  "Cell10_Temperature"
  Demux2/7 -> Gain20/1
  Demux2/6 -> Gain19/1
  Demux2/5 -> Gain18/1
  Gain21/1 -> Terminator44/1  "Cell5_Temperature"
  Rate Transition3/1 -> Celsius_to_Kelvin/1(K)
  Demux2/8 -> Gain21/1
  Gain18/1 -> Terminator43/1  "Cell8_Temperature"
  Gain15/1 -> Terminator48/1  "Cell1_Temperature"
  Gain23/1 -> Terminator46/1  "Cell3_Temperature"
  Celsius_to_Kelvin/1(C) -> Demux2/1
  Rate Transition6/1 -> Compare To Constant1/1  "Cell11_Current"
  Rate Transition4/1 -> Compare To Constant/1  "Cell12_Current"
  Rate Transition8/1 -> Compare To Constant3/1  "Cell9_Current"
  Rate Transition7/1 -> Compare To Constant2/1  "Cell10_Current"
  Compare To Constant/1 -> Terminator16/1  "Cell12_Bal_EN"
  Compare To Constant1/1 -> Terminator17/1  "Cell11_Bal_EN"
  Compare To Constant3/1 -> Terminator19/1  "Cell9_Bal_EN"
  Compare To Constant2/1 -> Terminator18/1  "Cell10_Bal_EN"
  Compare To Constant5/1 -> Terminator21/1  "Cell7_Bal_EN"
  Compare To Constant4/1 -> Terminator20/1  "Cell8_Bal_EN"
  Rate Transition10/1 -> Compare To Constant5/1  "Cell7_Current"
  Rate Transition12/1 -> Compare To Constant6/1  "Cell6_Current"
  Compare To Constant6/1 -> Terminator22/1  "Cell6_Bal_EN"
  Rate Transition9/1 -> Compare To Constant4/1  "Cell8_Current"
  Rate Transition13/1 -> Compare To Constant7/1  "Cell5_Current"
  Compare To Constant7/1 -> Terminator23/1  "Cell5_Bal_EN"
  Compare To Constant9/1 -> Terminator25/1  "Cell3_Bal_EN"
  Compare To Constant8/1 -> Terminator24/1  "Cell4_Bal_EN"
  Rate Transition15/1 -> Compare To Constant9/1  "Cell3_Current"
  Rate Transition16/1 -> Compare To Constant10/1  "Cell2_Current"
  Compare To Constant10/1 -> Terminator26/1  "Cell2_Bal_EN"
  Rate Transition14/1 -> Compare To Constant8/1  "Cell4_Current"
  Rate Transition11/1 -> Compare To Constant11/1  "Cell1_Current"
  Compare To Constant11/1 -> Terminator27/1  "Cell1_Bal_EN"
  Cells_SOCs/1 -> Rate Transition5/1
  Demux4/1 -> Gain36/1
  Demux4/2 -> Gain37/1
  Demux4/3 -> Gain38/1
  Demux4/4 -> Gain39/1
  Demux4/5 -> Gain40/1
  Demux4/6 -> Gain41/1
  Demux4/12 -> Gain47/1
  Demux4/11 -> Gain46/1
  Demux4/10 -> Gain45/1
  Demux4/9 -> Gain44/1
  Demux4/7 -> Gain42/1
  Demux4/8 -> Gain43/1
  Gain36/1 -> Terminator50/1  "Cell12_SOC"
  Gain37/1 -> Terminator51/1  "Cell11_SOC"
  Gain38/1 -> Terminator52/1  "Cell10_SOC"
  Gain39/1 -> Terminator53/1  "Cell9_SOC"
  Gain40/1 -> Terminator54/1  "Cell8_SOC"
  Gain41/1 -> Terminator55/1  "Cell7_SOC"
  Gain42/1 -> Terminator56/1  "Cell6_SOC"
  Gain43/1 -> Terminator57/1  "Cell5_SOC"
  Gain44/1 -> Terminator58/1  "Cell4_SOC"
  Gain45/1 -> Terminator59/1  "Cell3_SOC"
  Gain46/1 -> Terminator60/1  "Cell2_SOC"
  Gain47/1 -> Terminator61/1  "Cell1_SOC"
  Rate Transition5/1 -> Demux4/1, Sum of Elements/1
  Add/1 -> Terminator62/1  "Pack_Voltage"
  Open_Circuits_Value/1 -> Broken_Wires/1
  Short_Circuits_Value/1 -> Short-Circuits/1
  Demux5/1 -> Gain57/1  "SOC_CC"
  Demux5/2 -> Gain58/1  "SOC_UKF"
  Demux5/3 -> Gain59/1  "SOC_EKF"
  Max/1 -> Subtract/1
  Min/1 -> Subtract/2
  Subtract/1 -> Gain60/1
  Gain48/1 -> Terminator/1  "Discharge_Current_Limit"
  Gain49/1 -> Terminator3/1  "Charge_Current_Limit"
  Gain50/1 -> Terminator4/1  "Charge_Current_Req"
  Gain51/1 -> Terminator5/1  "Bal_Cmd"
  Gain52/1 -> Terminator8/1  "Overcurrent"
  Gain53/1 -> Terminator9/1  "HighTemp"
  Gain54/1 -> Terminator10/1  "LowTemp"
  Gain55/1 -> Terminator11/1  "OverVolt"
  Gain56/1 -> Terminator12/1  "LowVolt"
  Gain57/1 -> Terminator7/1  "SOC_CC"
  Gain59/1 -> Terminator64/1  "SOC_EKF"
  Bus Selector1/1 -> Bus Selector2/1  "<BMS_Faults>"
  Gain58/1 -> Terminator63/1  "SOC_UKF"
  Gain24/1 -> Median Filter/1
  Gain25/1 -> Median Filter1/1
  Gain26/1 -> Median Filter2/1
  Gain27/1 -> Median Filter3/1
  Gain28/1 -> Median Filter4/1
  Gain29/1 -> Median Filter5/1
  Gain32/1 -> Median Filter8/1
  Gain35/1 -> Median Filter11/1
  Gain30/1 -> Median Filter6/1
  Gain33/1 -> Median Filter9/1
  Gain34/1 -> Median Filter10/1
  Gain31/1 -> Median Filter7/1
  Gain60/1 -> Terminator65/1  "Charge Imbalance"
  Gain61/1 -> Demux/1
  Median Filter/1 -> Rate Transition4/1
  Median Filter1/1 -> Rate Transition6/1
  Median Filter2/1 -> Rate Transition7/1
  Median Filter3/1 -> Rate Transition8/1
  Median Filter4/1 -> Rate Transition9/1
  Median Filter5/1 -> Rate Transition10/1
  Median Filter6/1 -> Rate Transition12/1
  Median Filter7/1 -> Rate Transition13/1
  Median Filter8/1 -> Rate Transition14/1
  Median Filter9/1 -> Rate Transition15/1
  Median Filter10/1 -> Rate Transition16/1
  Median Filter11/1 -> Rate Transition11/1
  Gain62/1 -> Terminator14/1  "Pack Current"
  Sum of Elements/1 -> Gain63/1
  Gain63/1 -> Terminator66/1  "SOC"

== system SystemModel/BMS/HIL/Controller/PLANT-Rx ==
  "CAN Read " : speedgoatlib_IO611/CAN Read   moduleType=IO611  id=1  channel=2  canType=CAN (HS)  useBusOut=off  HasMulRead=Single Read from Buffer (FIFO)  MsgIDlist=[1 2]  isEFF=off  LabelInHex=on  enableInput=off  ts=-1  initValues=[611 1 -1 1 1 1 0 0 0 1 2 1 2]
      settings: SourceProductName=IO611
  Data Type Conversion{,1..3} (4 alike) : DataTypeConversion  OutDataTypeStr=single  SaturateOnIntegerOverflow=off  RndMeth=Floor
  Messages : Subsystem
  While Iterator : WhileIterator  MaxIters=-1  WhileBlockType=do-while
  BMS_Faults : Outport
  Charging_State : Outport  Port=2
  BMS_State : Outport  Port=3
  SOC : Outport  Port=4
  Discharge_Current_Limit : Outport  Port=5
  Charge_Current_Limit : Outport  Port=6
  Charge_Current_Req : Outport  Port=7
  wires:
  "CAN Read "/2 -> Messages/4(ID_0x502), Messages/3(ID_0x501), Messages/2(ID_0x202), Messages/1(ID_0x201)
  "CAN Read "/1 -> While Iterator/1
  Messages/1(Discharge_Current_Limit) -> Data Type Conversion/1
  Messages/7(Charging_State) -> Charging_State/1
  Messages/2(Charge_Current_Limit) -> Data Type Conversion1/1
  Messages/3(Charge_Current_Req) -> Data Type Conversion2/1
  Messages/4(SOC) -> Data Type Conversion3/1
  Messages/6(BMS_State) -> BMS_State/1
  Data Type Conversion/1 -> Discharge_Current_Limit/1
  Data Type Conversion1/1 -> Charge_Current_Limit/1
  Data Type Conversion2/1 -> Charge_Current_Req/1
  Data Type Conversion3/1 -> SOC/1
  Messages/5(BMS_Faults) -> BMS_Faults/1

== system SystemModel/BMS/HIL/Controller/PLANT-Tx ==
  to_Controller : Inport
  to_Controller_SRE : Inport  Port=2
  12-Cell : Subsystem  VariantControl=Ns_Module == 12
  wires:
  to_Controller/1 -> 12-Cell/1(to_Controller)
  to_Controller_SRE/1 -> 12-Cell/2(to_Controller_SRE)

== system SystemModel/BMS/MIL/Cell Monitoring Unit/Balancing_Circuit ==
  Bal_Cmd_Controller : Inport
  12-Cell : Subsystem  VariantControl=Ns_Module == 12
  Cells : PMIOPort  Side=Left
  Balancing_Currents : Outport
  wires:
  Bal_Cmd_Controller/1 -> 12-Cell/1(Bal_Cmd_Controller)
  12-Cell/1(Balancing_Currents) -> Balancing_Currents/1
  connections:
  Cells/RConn1 -- 12-Cell/LConn1

== system SystemModel/BMS/MIL/Controller/BMS State Machine ==
  Discharge_Current_Limit : Inport
  Charge_Current_Limit : Inport  Port=2
  State_Request : Inport  Port=3  OutDataTypeStr=Enum: SRE
  Sensor_Values : Inport  Port=4
  Fault_Reset_Enable : Inport  Port=5
  Bus Selector : BusSelector  OutputSignals=Cell_Voltages,Pack_Voltage,Cell_Temperatures,Pack_Current
  Data Type Conversion : DataTypeConversion  OutDataTypeStr=boolean  SaturateOnIntegerOverflow=off  RndMeth=Floor
  State_Machine : Stateflow chart  TreatAsAtomicUnit=on  VariantControl=(default)
  Charge_Current_Req : Outport  OutMin=-100  OutMax=100  OutDataTypeStr=single  VectorParamsAs1DForOutWhenUnconnected=off
  Faults : Outport  Port=2  OutDataTypeStr=Bus: Faults  VectorParamsAs1DForOutWhenUnconnected=off  BusOutputAsStruct=on
  Charging_State : Outport  Port=3
  BMS_State : Outport  Port=4  OutDataTypeStr=Enum: BMS_Controller_State  VectorParamsAs1DForOutWhenUnconnected=off
  wires:
  State_Machine/2(Fault_out) -> Faults/1  "Faults"
  Bus Selector/1 -> State_Machine/4(Cell_Voltages)  "<Cell_Voltages>"
  State_Machine/1(ChargeCurrentReq) -> Charge_Current_Req/1  "Charge_Current_Req"
  State_Request/1 -> State_Machine/3(State_Request)
  Discharge_Current_Limit/1 -> State_Machine/1(DischargeCurrentLimit)
  Charge_Current_Limit/1 -> State_Machine/2(ChargeCurrentLimit)
  Bus Selector/3 -> State_Machine/6(Cell_Temperatures)  "<Cell_Temperatures>"
  Bus Selector/2 -> State_Machine/5(Pack_Voltage)  "<Pack_Voltage>"
  Bus Selector/4 -> State_Machine/7(Pack_Current)  "<Pack_Current>"
  Sensor_Values/1 -> Bus Selector/1
  Fault_Reset_Enable/1 -> Data Type Conversion/1
  Data Type Conversion/1 -> State_Machine/8(Fault_Reset_Enable)
  State_Machine/3(ChargeModeReq) -> Charging_State/1  "Charging_State"
  State_Machine/4(BMS_State) -> BMS_State/1  "BMS_State"

== system SystemModel/BMS/MIL/Controller/Balancing Logic ==
  BMS_State : Inport  OutDataTypeStr=Enum: BMS_Controller_State  PortDimensions=1
  Sensor_Values : Inport  Port=2
  Balancing : Stateflow chart  TreatAsAtomicUnit=on  VariantControl=(default)
  Bus Selector1 : BusSelector  OutputSignals=Cell_Voltages
  Bal_Cmd : Outport  OutDataTypeStr=boolean  PortDimensions=[1,NumModules*Ns_Module]  VectorParamsAs1DForOutWhenUnconnected=off
  wires:
  Balancing/1(Bal_Cmd) -> Bal_Cmd/1  "Bal_Cmd"
  Bus Selector1/1 -> Balancing/2(CellVoltages)  "<Cell_Voltages>"
  Sensor_Values/1 -> Bus Selector1/1
  BMS_State/1 -> Balancing/1(BMS_State)

== system SystemModel/BMS/MIL/Controller/Current Calculations ==
  BMS_Input : Inport
  Bus Selector : BusSelector  OutputSignals=Cell_Voltages,Cell_Temperatures
  Charge_Current_Limit_Calc : Subsystem
  Discharge_Current_Limit_Calc : Subsystem
  MinMax : MinMax
  MinMax1 : MinMax
  MinMax2 : MinMax  Function=max
  MinMax4 : MinMax  Function=max
  Discharge_Current_Limit : Outport
  Charge_Current_Limit : Outport  Port=2
  wires:
  MinMax/1 -> Discharge_Current_Limit_Calc/1(MinCellVolt)  "Min_Cell_Volt"
  MinMax4/1 -> Discharge_Current_Limit_Calc/3(MaxCellTemp), Charge_Current_Limit_Calc/3(MaxCellTemp)  "Max_Cell_Temp"
  MinMax1/1 -> Discharge_Current_Limit_Calc/2(MinCellTemp), Charge_Current_Limit_Calc/2(MinCellTemp)  "Min_Cell_Temp"
  MinMax2/1 -> Charge_Current_Limit_Calc/1(MaxCellVolt)  "Max_Cell_Volt"
  Discharge_Current_Limit_Calc/1(Discharge_Current_Limit) -> Discharge_Current_Limit/1  "Discharge_Current_Limit"
  Charge_Current_Limit_Calc/1(Charge_Current_Limit) -> Charge_Current_Limit/1  "Charge_Current_Limit"
  Bus Selector/1 -> MinMax/1, MinMax2/1  "<Cell_Voltages>"
  Bus Selector/2 -> MinMax4/1, MinMax1/1  "<Cell_Temperatures>"
  BMS_Input/1 -> Bus Selector/1

== system SystemModel/BMS/MIL/Controller/SOC Calculation ==
  BMS_State : Inport  OutDataTypeStr=Enum: BMS_Controller_State
  Sensor_Values : Inport  Port=2
  Bus Selector2 : BusSelector  OutputSignals=Pack_Current,Cell_Voltages,Cell_Temperatures
  Compare To Constant : simulink/Logic and Bit Operations/Compare To Constant  relop=~=  const=BMS_Controller_State.BMS_Fault  OutDataTypeStr=boolean
  Coulomb Counting : Subsystem  VariantControl=SocAlgo==1
  Gain : Gain  Gain=100
  Measurement Function : Subsystem  TreatAsAtomicUnit=on
  Mux : Mux  Inputs=3
  PackCurrent : Gain  Gain=-1
  State Transition Function : Subsystem  TreatAsAtomicUnit=on
  Temp : Selector  InputPortWidth=Ns_Module*NumModules  IndexOptions=Index vector (dialog)  Indices=1  OutputSizes=1
  UKF_EKF_1TC : Subsystem  VariantControl=CellType==1
  Volt : Selector  InputPortWidth=Ns_Module*NumModules  IndexOptions=Index vector (dialog)  Indices=1  OutputSizes=1
  SOC : Outport  OutDataTypeStr=single  VectorParamsAs1DForOutWhenUnconnected=off
  wires:
  Mux/1 -> Gain/1  "SOC"
  UKF_EKF_1TC/1(SOC_UKF) -> Mux/2  "SOC_UKF"
  BMS_State/1 -> Compare To Constant/1
  Coulomb Counting/1(SOC) -> Mux/1  "SOC_CC"
  Volt/1 -> UKF_EKF_1TC/1(Cell_Voltage)
  Temp/1 -> Coulomb Counting/2(Temp), State Transition Function/2(Temperature K), Measurement Function/2(Temperature (K))
  Compare To Constant/1 -> UKF_EKF_1TC/Enable
  UKF_EKF_1TC/2(SOC_EKF) -> Mux/3  "SOC_EKF"
  Bus Selector2/1 -> Coulomb Counting/1(Curr), PackCurrent/1  "<Pack_Current>"
  PackCurrent/1 -> State Transition Function/1(Current), Measurement Function/1(Current)  "PackCurrent"
  Bus Selector2/3 -> Temp/1  "<Cell_Temperatures>"
  Bus Selector2/2 -> Volt/1  "<Cell_Voltages>"
  Sensor_Values/1 -> Bus Selector2/1
  Gain/1 -> SOC/1
